simulink model "sim_NONLINEAR_2DOF"  (R2021b)
settings: Solver=VariableStepAuto  StartTime=0.0  StopTime=Ts  MaxStep=1e-03  RelTol=1e-3
values from neighbouring files (symbols this model uses):
  choice2 = menu('Road profile h','Step signal h0 = 5cm','Sinewave','Chirp')    [ES_2DOF_ANIM_TF.m]
  F_NL_damp = 4*[-672 -493 -450 -400 -351 -199 0 301 1068 1260 1386 1514 2130]    [ES_2DOF_ANIM_TF.m]
  f_sampling = 1*10^3    (= 1000)    [Dati_Necessari.m]    (also in ES_2DOF_ANIM_TF.m)
  H = [0 k1p]'    [Dati_Necessari.m]    (also in ES2_2DOF.m; ES_2DOF_ANIM_TF.m)
  h = 5/100    (= 0.05)    [Dati_Necessari.m]    (also in ES_2DOF_ANIM_TF.m)
  h0 = 2/100    (= 0.02)    [Dati_Necessari.m]    (also in ES01_Comfort_4dof_stud.m = 0.01; ES_2DOF_ANIM_TF.m)
  K = [k -k; -k k+k1p]    [Dati_Necessari.m]    (also in ES2_2DOF.m = [k -k; ES_2DOF_ANIM_TF.m = [k -k)
  lambda = 2    [Dati_Necessari.m]    (also in ES01_Comfort_4dof_stud.m = 2*pi*V./OM; ES_2DOF_ANIM_TF.m)
  M = [ms 0; 0 mu]    [Dati_Necessari.m]    (also in ES2_2DOF.m = [ms 0; ES_2DOF_ANIM_TF.m = [ms 0)
  slope = h/0.01    (= 5)    [Dati_Necessari.m]    (also in ES_2DOF_ANIM_TF.m)
  Ts = 4    [DatiSospensione.m]    (also in ES_2DOF_ANIM_TF.m = 100)
  v = 0    [Dati_Necessari.m]    (also in ES_2DOF_ANIM_TF.m = 36.1111111111)
  v_NL_damp = [-1000 -520 -390 -260 -130 -50 0 50 130 260 390 520 1000]/1000    [ES_2DOF_ANIM_TF.m]
  z0 = 0    [Dati_Necessari.m]    (also in ES_2DOF_ANIM_TF.m)
  zd0 = 0    [Dati_Necessari.m]    (also in ES_2DOF_ANIM_TF.m)
libraries: simulink x2
settings Model: Creator=Utente  LastModifiedBy=Utente
settings DataIOCC: ReturnWorkspaceOutputs=off

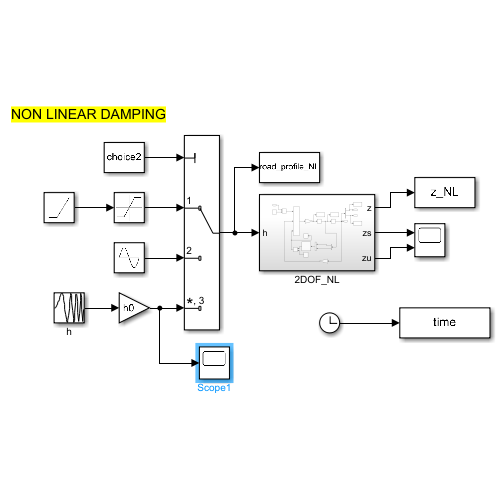
[thumbnail: Simulink's stored preview of the top-level diagram]
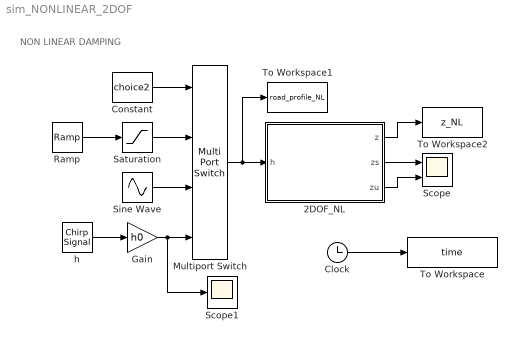
== system sim_NONLINEAR_2DOF ==
  note: NON LINEAR DAMPING
  2DOF_NL : Subsystem
  Clock : Clock
  Constant : Constant  Value=choice2
  Gain : Gain  Gain=h0
  Multiport Switch : MultiPortSwitch
  Ramp : simulink/Sources/Ramp  slope=slope  start=0.01  InitialOutput=0
  Saturation : Saturate  UpperLimit=h
  Scope : Scope  NumInputPorts=2
  Scope1 : Scope
  Sine Wave : Sin  Amplitude=h0  Frequency=2*pi*v/lambda  SampleTime=0
  To Workspace : ToWorkspace  VariableName=time  SampleTime=1/f_sampling
  To Workspace1 : ToWorkspace  VariableName=road_profile_NL  SampleTime=1/f_sampling
      settings: Decimation=decimation
  To Workspace2 : ToWorkspace  VariableName=z_NL  SampleTime=1/f_sampling
  h : simulink/Sources/Chirp Signal  f1=f_in  T=Ts  f2=f_end
  wires:
  Sine Wave/1 -> Multiport Switch/3
  Saturation/1 -> Multiport Switch/2
  2DOF_NL/1(z) -> To Workspace2/1
  Ramp/1 -> Saturation/1
  2DOF_NL/3(zu) -> Scope/2
  Multiport Switch/1 -> 2DOF_NL/1(h), To Workspace1/1
  Constant/1 -> Multiport Switch/1
  2DOF_NL/2(zs) -> Scope/1
  Clock/1 -> To Workspace/1
  h/1 -> Gain/1
  Gain/1 -> Scope1/1, Multiport Switch/4

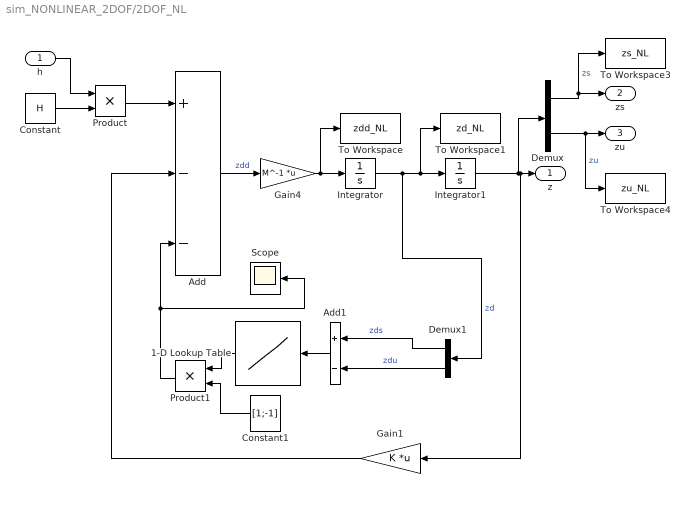
== system sim_NONLINEAR_2DOF/2DOF_NL ==
  h : Inport
  1-D Lookup Table : Lookup_n-D  NumberOfTableDimensions=1  BreakpointsForDimension1=v_NL_damp  Table=F_NL_damp  InternalRulePriority=Speed  RndMeth=Simplest  InputSameDT=on
  Add : Sum  Inputs=+--
  Add1 : Sum  Inputs=+-
  Constant : Constant  Value=H
  Constant1 : Constant  Value=[1;-1]
  Demux : Demux  Outputs=2
  Demux1 : Demux  Outputs=2
  Gain1 : Gain  Gain=K  Multiplication=Matrix(K*u)
  Gain4 : Gain  Gain=M^-1  Multiplication=Matrix(K*u)
  Integrator : Integrator  InitialCondition=zd0
  Integrator1 : Integrator  InitialCondition=z0
  Product : Product
  Product1 : Product
  Scope : Scope
  To Workspace : ToWorkspace  VariableName=zdd_NL  SaveFormat=Timeseries  SampleTime=1/f_sampling
  To Workspace1 : ToWorkspace  VariableName=zd_NL  SaveFormat=Timeseries  SampleTime=1/f_sampling
  To Workspace3 : ToWorkspace  VariableName=zs_NL  SampleTime=1/f_sampling
  To Workspace4 : ToWorkspace  VariableName=zu_NL  SampleTime=1/f_sampling
  z : Outport
  zs : Outport  Port=2
  zu : Outport  Port=3
  wires:
  h/1 -> Product/1
  Add/1 -> Gain4/1  "zdd"
  Integrator/1 -> Demux1/1, Integrator1/1, To Workspace1/1  "zd"
  Integrator1/1 -> Gain1/1, z/1, Demux/1
  Demux/1 -> zs/1, To Workspace3/1  "zs"
  Demux/2 -> zu/1, To Workspace4/1  "zu"
  Constant/1 -> Product/2
  Product/1 -> Add/1
  Gain4/1 -> Integrator/1, To Workspace/1
  Demux1/1 -> Add1/1  "zds"
  Demux1/2 -> Add1/2  "zdu"
  Add1/1 -> 1-D Lookup Table/1
  1-D Lookup Table/1 -> Product1/1
  Constant1/1 -> Product1/2
  Product1/1 -> Add/3, Scope/1
  Gain1/1 -> Add/2
